simulink model "PMotorTemperatureDerate"  (R2024b)
settings: Solver=FixedStepDiscrete  StartTime=0.0  StopTime=1  FixedStep=0.001  RelTol=1e-3  EnableMultiTasking=on
settings Model: DataDictionary=Master_Dictionary.sldd  EnableAccessToBaseWorkspace=off  Creator=torni  LastModifiedBy=oxbro
settings SolverCC: AlgebraicLoopSolver=TrustRegion
settings DataIOCC: ReturnWorkspaceOutputs=off
settings OptimizationCC: DefaultParameterBehavior=Inlined  EnhancedBackFolding=on  PassReuseOutputArgsAs=Individual arguments  ZeroExternalMemoryAtStartup=off  ZeroInternalMemoryAtStartup=off  MaxStackSize=512  OptimizeBlockOrder=speed  DifferentSizesBufferReuse=on  OptimizationCustomize=off  EfficientTunableParamExpr=on
settings DebuggingCC: ParameterTunabilityLossMsg=error  UnconnectedInputMsg=warning  UnconnectedOutputMsg=warning  UnconnectedLineMsg=warning  ArithmeticOperatorsInVariantConditions=warning
settings HardwareCC: ProdBitPerPointer=32  ProdBitPerSizeT=32  ProdBitPerPtrDiffT=32  ProdLargestAtomicInteger=Long  ProdLargestAtomicFloat=Double  ProdWordSize=32  ProdLongLongMode=on  ProdHWDeviceType=ARM Compatible->ARM Cortex-M
settings ModelReferenceCC: EnableRefExpFcnMdlSchedulingChecks=on
settings SFSimCC: MATLABDynamicMemAlloc=off  CustomCodeUndefinedFunction=UseInterfaceOnly
settings RTWCC: Description=Embedded Coder  SystemTargetFile=ert.tlc  HardwareBoard=STM32H7xx Based (Single-core)  TemplateMakefile=ert_default_tmf  CustomHeaderCode="#include \"stm32h7xx_ll_tim.h\""  CustomInitializer=LL_TIM_EnableCounter(TIM2);  Toolchain=GNU Tools for ARM Embedded Processors  GPUComputeCapability=3.5
settings CodeAppCC: ForceParamTrailComments=on  IgnoreCustomStorageClasses=off  OperatorAnnotations=on  SimulinkDataObjDesc=on  SFDataObjDesc=on  InsertBlockDesc=on
settings ERTTargetCC: TargetLangStandard=C99 (ISO)  CodeReplacementLibrary=ARM Cortex-M  ExtModeTransport=3  ExtModeStaticAlloc=on  ExtModeStaticAllocSize=2048  ExtModeMexFile=ext_xcp  ExtModeIntrfLevel=Level2 - Open

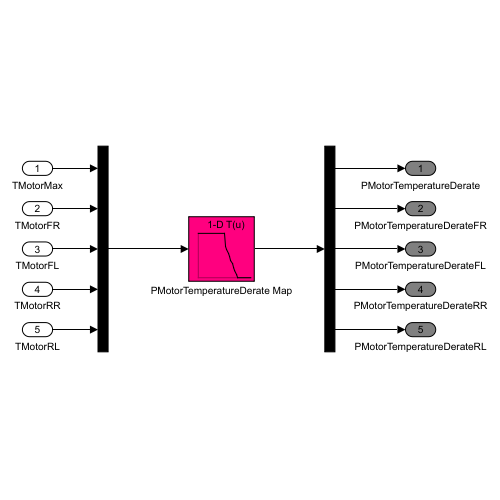
[thumbnail: Simulink's stored preview of the top-level diagram]
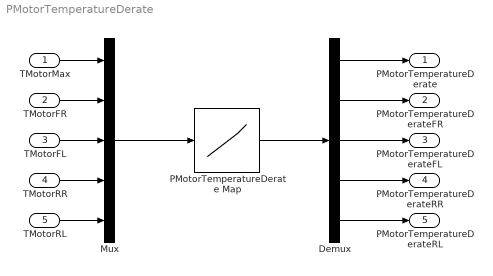
== system PMotorTemperatureDerate ==
  "TMotorMax " : Inport  OutDataTypeStr=double
  TMotorFR : Inport  Port=2  OutDataTypeStr=double
  TMotorFL : Inport  Port=3  OutDataTypeStr=double
  TMotorRR : Inport  Port=4  OutDataTypeStr=double
  TMotorRL : Inport  Port=5  OutDataTypeStr=double
  Demux : Demux  Outputs=5
  Mux : Mux  Inputs=5
  PMotorTemperatureDerate Map : Lookup_n-D  NumberOfTableDimensions=1  BreakpointsForDimension1=[0,100,105,110,115,120,125,130,135,140,145,150,200]  Table=[100,100,70.2,62.4,54.6,46.8,39,31.2,23.4,15.6,7.8,0,0]  InternalRulePriority=Speed  RndMeth=Simplest
  PMotorTemperatureDerate : Outport  OutDataTypeStr=double  VectorParamsAs1DForOutWhenUnconnected=off
  PMotorTemperatureDerateFR : Outport  Port=2  OutDataTypeStr=double  VectorParamsAs1DForOutWhenUnconnected=off
  PMotorTemperatureDerateFL : Outport  Port=3  OutDataTypeStr=double  VectorParamsAs1DForOutWhenUnconnected=off
  PMotorTemperatureDerateRR : Outport  Port=4  OutDataTypeStr=double  VectorParamsAs1DForOutWhenUnconnected=off
  PMotorTemperatureDerateRL : Outport  Port=5  OutDataTypeStr=double  VectorParamsAs1DForOutWhenUnconnected=off
  wires:
  TMotorFL/1 -> Mux/3
  TMotorFR/1 -> Mux/2
  "TMotorMax "/1 -> Mux/1
  Demux/1 -> PMotorTemperatureDerate/1
  Demux/5 -> PMotorTemperatureDerateRL/1
  Mux/1 -> PMotorTemperatureDerate Map/1
  Demux/3 -> PMotorTemperatureDerateFL/1
  Demux/4 -> PMotorTemperatureDerateRR/1
  TMotorRR/1 -> Mux/4
  PMotorTemperatureDerate Map/1 -> Demux/1
  Demux/2 -> PMotorTemperatureDerateFR/1
  TMotorRL/1 -> Mux/5
